simulink library "Power_Shaft3_Electric_A1_L2_R2"  (R2022b)
settings: Solver=VariableStepAuto  StartTime=0.0  StopTime=10.0  RelTol=1e-3
undefined symbols (not defined in the file): ShaftA1, ShaftL2, ShaftR2, VDatabase
libraries: Power_Components x4, fl_lib x2, sm_lib x1, Cooling_Motor3 x1
Description:
  | Component of Simscape Vehicle Templates Library
  | 
  | Copyright 2018-2024 The MathWorks, Inc.
settings Model: Creator=smiller  LastModifiedBy=smiller
settings SolverCC: AlgebraicLoopSolver=TrustRegion
settings DataIOCC: ReturnWorkspaceOutputs=off
settings DebuggingCC: UnconnectedInputMsg=warning  UnconnectedOutputMsg=warning  UnconnectedLineMsg=warning  SFMachineParentedDataDiag=warning  ArithmeticOperatorsInVariantConditions=warning
settings ModelReferenceCC: EnableRefExpFcnMdlSchedulingChecks=on
settings SFSimCC: CustomCodeUndefinedFunction=UseInterfaceOnly
settings RTWCC: DLArmComputeVersion=19.05

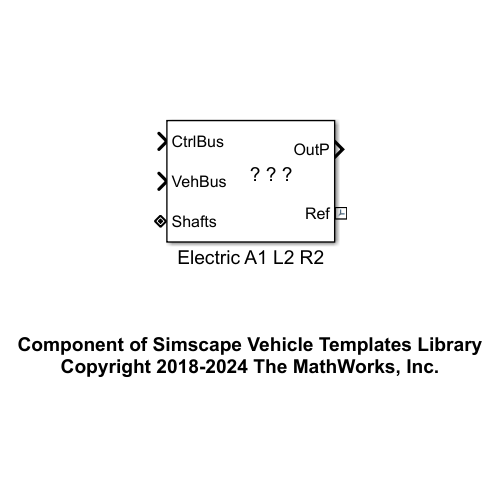
[thumbnail: Simulink's stored preview of the top-level diagram]
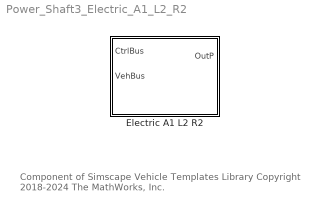
== system Power_Shaft3_Electric_A1_L2_R2 ==
  note: Component of Simscape Vehicle Templates Library
      | Copyright 2018-2024 The MathWorks, Inc.
  Electric A1 L2 R2 : Subsystem  mask(Electric Propulsion with Three Motors){Power=VDatabase.Power.Electric3Motor_A1_L2_R2_default}
      mask prompts: Power "Power 3 Motor (structure)"
      mask help: Three electric motors with optional cooling system. Physical connections for the three motor shafts are in bus Shafts.
      mask Display: image('sm_car_vehicle_power_e3motor_A1L2R2_IMAGE.png');

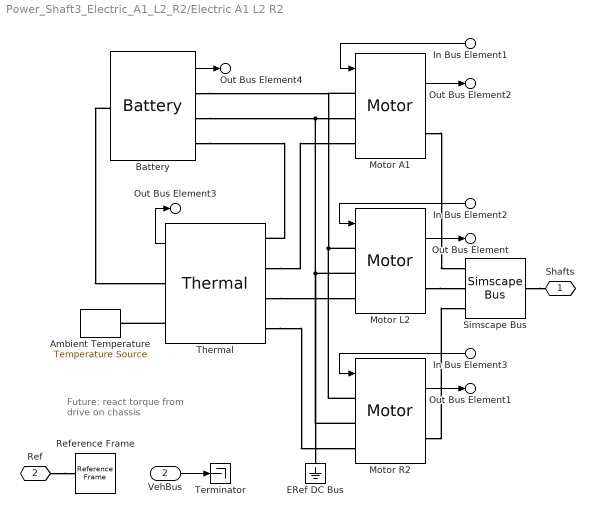
== system Power_Shaft3_Electric_A1_L2_R2/Electric A1 L2 R2 ==
  note: Future:
      | react torque
      | from drive
      | on chassis
  In Bus Element1 : Inport  PortName=CtrlBus  Element=MMotorA1Demand
  In Bus Element2 : Inport  PortName=CtrlBus  Element=MMotorL2Demand
  In Bus Element3 : Inport  PortName=CtrlBus  Element=MMotorR2Demand
  VehBus : Inport  Port=2
  Ambient Temperature : fl_lib/Thermal/Thermal Sources/Temperature Source  temperature=Power.TAmbient.Value K
  Battery : Power_Components/Battery  SystemSampleTime=-1  VariantActivationTime=update diagram  Latency=0  AutoFrameSizeCalculation=off
  ERef DC Bus : fl_lib/Electrical/Electrical Elements/Electrical Reference
  Motor A1 : Power_Components/Motor  Motor=Power.MotorA1
  Motor L2 : Power_Components/Motor  Motor=Power.MotorL2
  Motor R2 : Power_Components/Motor  Motor=Power.MotorL2
  Reference Frame : sm_lib/Frames and Transforms/Reference Frame
  Simscape Bus : SimscapeBus  HierarchyStrings=ShaftA1;ShaftL2;ShaftR2
  Terminator : Terminator
  Thermal : Cooling_Motor3/Thermal  VariantControl=Variant1  LabelModeActiveChoice=None  VariantLabel=Power.Cooling.class.Value
      settings: AttributesFormatString=%<ActiveVariant>
  Shafts : PMIOPort  Side=Left
  Ref : PMIOPort  Port=2  Side=Right
  Out Bus Element : Outport  VectorParamsAs1DForOutWhenUnconnected=off  PortName=OutP  Element=MotorL2
  Out Bus Element1 : Outport  VectorParamsAs1DForOutWhenUnconnected=off  PortName=OutP  Element=MotorR2
  Out Bus Element2 : Outport  VectorParamsAs1DForOutWhenUnconnected=off  PortName=OutP  Element=MotorA1
  Out Bus Element3 : Outport  VectorParamsAs1DForOutWhenUnconnected=off  PortName=OutP  Element=Thermal
  Out Bus Element4 : Outport  VectorParamsAs1DForOutWhenUnconnected=off  PortName=OutP  Element=Battery
  wires:
  In Bus Element2/1 -> Motor L2/1
  In Bus Element1/1 -> Motor A1/1
  Motor L2/1 -> Out Bus Element/1
  Motor R2/1 -> Out Bus Element1/1
  Motor A1/1 -> Out Bus Element2/1
  In Bus Element3/1 -> Motor R2/1
  Thermal/1 -> Out Bus Element3/1
  VehBus/1 -> Terminator/1
  Battery/1 -> Out Bus Element4/1
  connections:
  Motor R2/RConn1 -- Simscape Bus/LConn3
  Motor L2/LConn2 -- Motor R2/LConn2 -- ERef DC Bus/LConn1 -- Battery/RConn2 -- Motor A1/LConn2
  Motor L2/LConn1 -- Battery/RConn1 -- Motor A1/LConn1 -- Motor R2/LConn1
  Motor A1/RConn1 -- Simscape Bus/LConn1
  Motor L2/RConn1 -- Simscape Bus/LConn2
  Simscape Bus/RConn1 -- Shafts/RConn1
  Ref/RConn1 -- Reference Frame/RConn1
  Thermal/LConn2 -- Motor A1/LConn3
  Thermal/LConn3 -- Motor L2/LConn3
  Thermal/LConn4 -- Motor R2/LConn3
  Thermal/RConn2 -- Ambient Temperature/LConn1
  Battery/RConn3 -- Thermal/LConn1
  Battery/LConn1 -- Thermal/RConn1
